simulink model "QP_9B_SimModel"  (R2014a)
settings: Solver=ode45  StartTime=0.0  StopTime=0.2  RelTol=1e-3
values from neighbouring files (symbols this model uses):
  B = mod(B, modulo)    [QP_MD5.m]    (also in QP_SolvePowerFlowEps.m = imag(Y))
  D = generator(:,GEN_D)    [QP_9B_RunModel.m]    (also in QP_MD5.m = C; QP_SimulateSystem.m; QP_SmallSignal.m = generator(:,GEN_D) .* generator(:,3)/100)
  delta0 = deltaState    [QP_9B_RunModel.m]    (also in QP_EXP_SimulateSystem.m = delta1(end,:)'; QP_SimulateSystem.m = delta0'; QP_SmallSignal.m = delta)
  E0_delta = delta0    [QP_9B_RunModel.m]
  G = ss(A, B, C, D)    [QP_HankelSV.m]    (also in QP_SolvePowerFlowEps.m = real(Y))
  H = generator(:,GEN_H)    [QP_9B_RunModel.m]    (also in QP_EXP_MultipleFiltering.m = 0.1; QP_SimulateSystem.m; QP_SmallSignal.m = generator(:,GEN_H) .* generator(:,3)/100)
  Pm = zeros(N_gen,1)    [QP_ClassicalEquilibrium.m]    (also in QP_ClassicalModel.m = [P;zeros(N_node - N_gen, 1)]; QP_SmallSignal.m = P0; QP_dw.m = [P;zeros(N_node - N_gen, 1)])
  RC_State0 = [RC_State.Data(end,1:StateIndex(faultyLine)-1),         RC_State.Data(end,StateIndex(faultyLine)+1:end)]    [QP_9B_RunModel.m]
  SysA = A_PostFault    [QP_9B_RunModel.m]    (also in QP_9B_SSModel.m = SysA([1:RM_State-1,RM_State+1:end],         [1:RM_State-1,RM; QP_ElectricNetwork.m = SysA([1:faultyBus-1, faultyBus+1:end],         [1:faultyBus-; QP_SmallSignal.m = SysA(2:end,2:end))
  SysB = B_PostFault    [QP_9B_RunModel.m]    (also in QP_9B_SSModel.m = SysB([1:RM_State-1,RM_State+1:end],:); QP_ElectricNetwork.m = SysB([1:faultyBus-1, faultyBus+1:end],:))
  SysC = C_PostFault    [QP_9B_RunModel.m]    (also in QP_9B_SSModel.m = SysC(:,[1:RM_State-1,RM_State+1:end]); QP_ElectricNetwork.m = SysC(:,[1:faultyBus-1, faultyBus+1:end]))
  w0 = omegaState    [QP_9B_RunModel.m]    (also in QP_SmallSignal.m = omega)
  XNoisePWR = statePWR([1:StateIndex(faultyLine)-1,              StateIndex(faultyLine)+1:end]) * PWR    [QP_9B_RunModel.m]
  YNoisePWR = outputPWR * PWR    [QP_9B_RunModel.m]
undefined symbols (not defined in the file or in its folder): magnitude
settings Model: Creator=Qiu  LastModifiedBy=qqin
settings DebuggingCC: UnderspecifiedInitializationDetection=Classic  SolverPrmCheckMsg=none  UnconnectedOutputMsg=none  StateNameClashWarn=warning

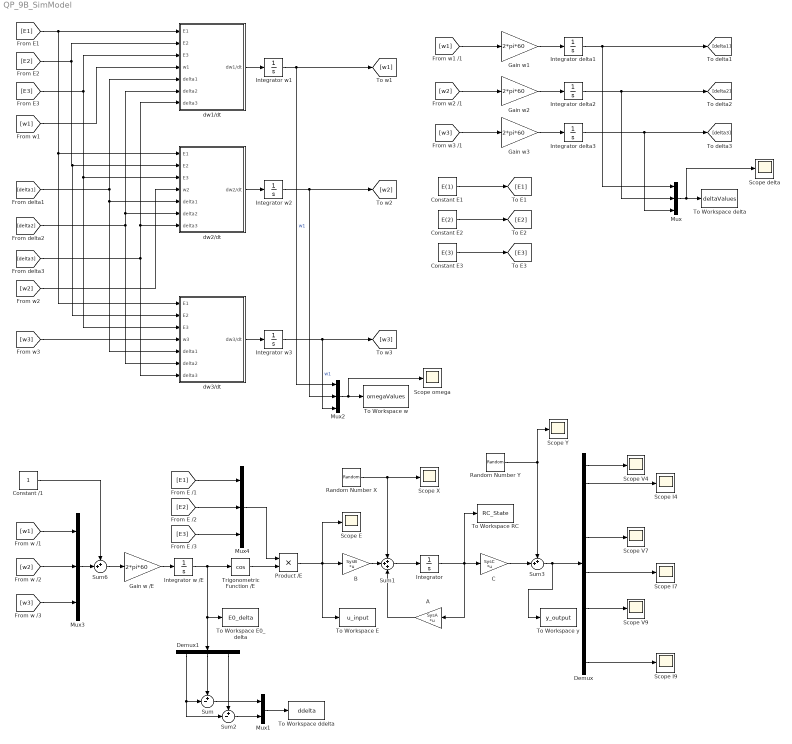
== system QP_9B_SimModel ==
  A : Gain  Gain=SysA  Multiplication=Matrix(K*u)
  B : Gain  Gain=SysB  Multiplication=Matrix(K*u)
  C : Gain  Gain=SysC  Multiplication=Matrix(K*u)
  Constant /1 : Constant
  Constant E1 : Constant  Value=E(1)
  Constant E2 : Constant  Value=E(2)
  Constant E3 : Constant  Value=E(3)
  Demux : Demux  Outputs=12
  Demux1 : Demux  Outputs=3
  Gain w /E : Gain  Gain=2*pi*60
  Gain w1 : Gain  Gain=2*pi*60
  Gain w2 : Gain  Gain=2*pi*60
  Gain w3 : Gain  Gain=2*pi*60
  Integrator : Integrator  InitialCondition=RC_State0
  Integrator delta1 : Integrator  InitialCondition=delta0(1)
  Integrator delta2 : Integrator  InitialCondition=delta0(2)
  Integrator delta3 : Integrator  InitialCondition=delta0(3)
  Integrator w /E : Integrator  InitialCondition=E0_delta
  Integrator w1 : Integrator  InitialCondition=w0(1)
  Integrator w2 : Integrator  InitialCondition=w0(2)
  Integrator w3 : Integrator  InitialCondition=w0(3)
  Mux{,2..4} (4 alike) : Mux  Inputs=3
  Mux1 : Mux  Inputs=2
  Product /E : Product
  Random Number X : RandomNumber  Variance=XNoisePWR  Seed=[round(rand(1)*10000)]  SampleTime=1/60/96
  Random Number Y : RandomNumber  Variance=YNoisePWR  Seed=[round(rand(1)*10000)]  SampleTime=1/60/96
  Scope E : Scope
      settings: MaxDataPoints=50000
  Scope I4 : Scope
      settings: SaveName=ScopeData6  MaxDataPoints=50000
  Scope I7 : Scope
      settings: SaveName=ScopeData7  MaxDataPoints=50000
  Scope I9 : Scope
      settings: SaveName=ScopeData8  MaxDataPoints=50000
  Scope V4 : Scope
      settings: MaxDataPoints=50000
  Scope V7 : Scope
      settings: SaveName=ScopeData2  MaxDataPoints=50000
  Scope V9 : Scope
      settings: SaveName=ScopeData3  MaxDataPoints=50000
  Scope X : Scope
      settings: SaveName=ScopeData10  MaxDataPoints=50000
  Scope Y : Scope
      settings: SaveName=ScopeData9  MaxDataPoints=50000
  Scope delta : Scope
      settings: SaveName=ScopeData4  MaxDataPoints=50000
  Scope omega : Scope
      settings: SaveName=ScopeData5  MaxDataPoints=50000
  Sum : Sum  Inputs=+-|
  Sum1 : Sum  Inputs=+++
  Sum2 : Sum  Inputs=+-|
  Sum3 : Sum  Inputs=++|
  Sum6 : Sum  Inputs=++|
  To Workspace E : ToWorkspace  VariableName=u_input  SaveFormat=Timeseries  SampleTime=-1
      settings: MaxDataPoints=Inf
  To Workspace E0_delta : ToWorkspace  VariableName=E0_delta  SampleTime=-1
      settings: MaxDataPoints=1
  To Workspace RC : ToWorkspace  VariableName=RC_State  SaveFormat=Timeseries  SampleTime=-1
      settings: MaxDataPoints=Inf
  To Workspace ddelta : ToWorkspace  VariableName=ddelta  SaveFormat=Timeseries  SampleTime=-1
      settings: MaxDataPoints=Inf
  To Workspace delta : ToWorkspace  VariableName=deltaValues  SampleTime=-1
      settings: MaxDataPoints=1
  To Workspace w : ToWorkspace  VariableName=omegaValues  SaveFormat=Timeseries  SampleTime=-1
      settings: MaxDataPoints=Inf
  To Workspace y : ToWorkspace  VariableName=y_output  SaveFormat=Timeseries  SampleTime=-1
      settings: MaxDataPoints=Inf
  Trigonometric Function /E : Trigonometry  Operator=cos
  dw1/dt : Subsystem
  dw2/dt : Subsystem
  dw3/dt : Subsystem
  wires:
  Integrator w1/1 -> Mux2/1, [w1]  "w1"
  Gain w1/1 -> Integrator delta1/1
  Integrator delta1/1 -> Mux/1, [delta1]
  [w1] -> Gain w1/1
  Gain w2/1 -> Integrator delta2/1
  [w2] -> Gain w2/1
  Gain w3/1 -> Integrator delta3/1
  [w3] -> Gain w3/1
  Integrator delta2/1 -> [delta2], Mux/2
  Integrator delta3/1 -> [delta3], Mux/3
  Constant E1/1 -> [E1]
  Constant E2/1 -> [E2]
  Constant E3/1 -> [E3]
  dw1/dt/1(dw1/dt) -> Integrator w1/1
  Integrator w2/1 -> Mux2/2, [w2]
  dw2/dt/1(dw2/dt) -> Integrator w2/1
  Integrator w3/1 -> Mux2/3, [w3]  "w1"
  dw3/dt/1(dw3/dt) -> Integrator w3/1
  Mux/1 -> Scope delta/1, To Workspace delta/1
  [w2] -> dw2/dt/4(w2)
  [w3] -> dw3/dt/4(w3)
  [E1] -> dw3/dt/1(E1), dw2/dt/1(E1), dw1/dt/1(E1)
  [E2] -> dw3/dt/2(E2), dw2/dt/2(E2), dw1/dt/2(E2)
  [E3] -> dw3/dt/3(E3), dw2/dt/3(E3), dw1/dt/3(E3)
  [delta1] -> dw1/dt/5(delta1), dw3/dt/5(delta1), dw2/dt/5(delta1)
  [delta2] -> dw3/dt/6(delta2), dw1/dt/6(delta2), dw2/dt/6(delta2)
  [delta3] -> dw3/dt/7(delta3), dw1/dt/7(delta3), dw2/dt/7(delta3)
  [w1] -> dw1/dt/4(w1)
  Mux2/1 -> Scope omega/1, To Workspace w/1
  Sum1/1 -> Integrator/1
  Integrator/1 -> To Workspace RC/1, A/1, C/1
  Product /E/1 -> To Workspace E/1, Scope E/1, B/1
  Demux/1 -> Scope V4/1
  Demux/5 -> Scope V7/1
  Demux/9 -> Scope V9/1
  Trigonometric Function /E/1 -> Product /E/2
  Integrator w /E/1 -> Demux1/1, To Workspace E0_delta/1, Trigonometric Function /E/1
  Constant /1/1 -> Sum6/1
  Sum6/1 -> Gain w /E/1
  Demux/2 -> Scope I4/1
  Demux/12 -> Scope I9/1
  Demux/7 -> Scope I7/1
  Gain w /E/1 -> Integrator w /E/1
  Mux3/1 -> Sum6/2
  [w1] -> Mux3/1
  [w2] -> Mux3/2
  [w3] -> Mux3/3
  [E1] -> Mux4/1
  [E2] -> Mux4/2
  [E3] -> Mux4/3
  Mux4/1 -> Product /E/1
  Demux1/1 -> Sum/2, Sum2/2
  Demux1/2 -> Sum/1
  Demux1/3 -> Sum2/1
  Mux1/1 -> To Workspace ddelta/1
  Sum/1 -> Mux1/1
  Sum2/1 -> Mux1/2
  B/1 -> Sum1/2
  A/1 -> Sum1/3
  Random Number X/1 -> Scope X/1, Sum1/1
  Random Number Y/1 -> Scope Y/1, Sum3/1
  C/1 -> Sum3/2
  Sum3/1 -> To Workspace y/1, Demux/1

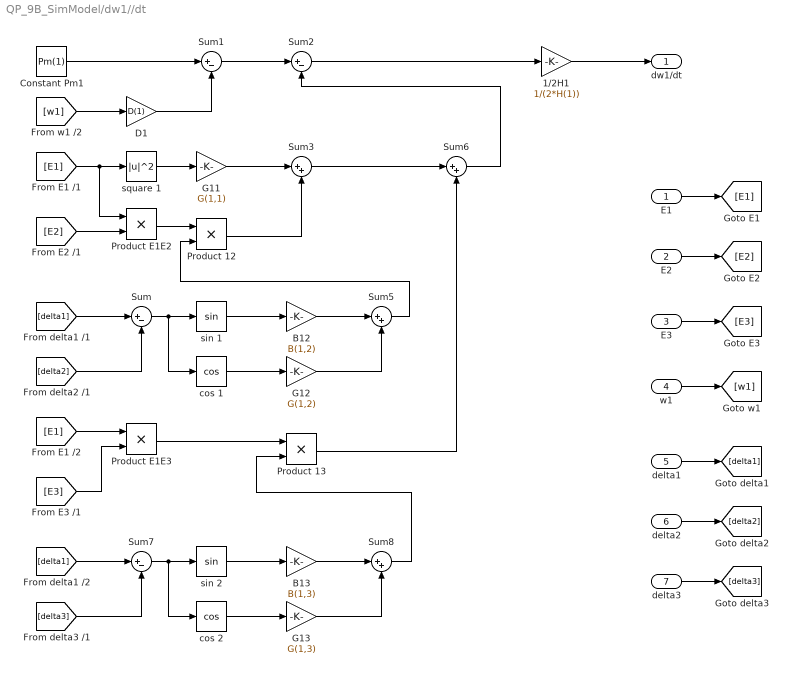
== system QP_9B_SimModel/dw1//dt ==
  E1 : Inport
  E2 : Inport  Port=2
  E3 : Inport  Port=3
  w1 : Inport  Port=4
  delta1 : Inport  Port=5
  delta2 : Inport  Port=6
  delta3 : Inport  Port=7
  1/2H1 : Gain  Gain=1/(2*H(1))
  B12 : Gain  Gain=B(1,2)
  B13 : Gain  Gain=B(1,3)
  Constant Pm1 : Constant  Value=Pm(1)
  D1 : Gain  Gain=D(1)
  G11 : Gain  Gain=G(1,1)
  G12 : Gain  Gain=G(1,2)
  G13 : Gain  Gain=G(1,3)
  Product 12 : Product
  Product 13 : Product
  Product E1E2 : Product
  Product E1E3 : Product
  Sum{,1..2,7} (4 alike) : Sum  Inputs=|+-
  Sum{3,5..6,8} (4 alike) : Sum  Inputs=|++
  cos 1 : Trigonometry  Operator=cos
  cos 2 : Trigonometry  Operator=cos
  sin 1 : Trigonometry
  sin 2 : Trigonometry
  square 1 : Math  Operator=magnitude^2  SaturateOnIntegerOverflow=on
  dw1/dt : Outport
  wires:
  G11/1 -> Sum3/1
  Sum3/1 -> Sum6/1
  Product 12/1 -> Sum3/2
  [delta2] -> Sum/2
  Product E1E2/1 -> Product 12/1
  sin 1/1 -> B12/1
  G12/1 -> Sum5/2
  [E2] -> Product E1E2/2
  [E1] -> Product E1E3/1
  B12/1 -> Sum5/1
  Sum8/1 -> Product 13/2
  Product 13/1 -> Sum6/2
  Sum2/1 -> 1/2H1/1
  Sum6/1 -> Sum2/2
  Sum7/1 -> cos 2/1, sin 2/1
  [delta1] -> Sum7/1
  sin 2/1 -> B13/1
  [delta3] -> Sum7/2
  cos 2/1 -> G13/1
  B13/1 -> Sum8/1
  G13/1 -> Sum8/2
  1/2H1/1 -> dw1/dt/1
  [delta1] -> Sum/1
  square 1/1 -> G11/1
  Constant Pm1/1 -> Sum1/1
  Sum1/1 -> Sum2/1
  D1/1 -> Sum1/2
  Product E1E3/1 -> Product 13/1
  Sum/1 -> cos 1/1, sin 1/1
  [E3] -> Product E1E3/2
  [w1] -> D1/1
  cos 1/1 -> G12/1
  [E1] -> Product E1E2/1, square 1/1
  Sum5/1 -> Product 12/2
  E1/1 -> [E1]
  E2/1 -> [E2]
  E3/1 -> [E3]
  w1/1 -> [w1]
  delta1/1 -> [delta1]
  delta2/1 -> [delta2]
  delta3/1 -> [delta3]

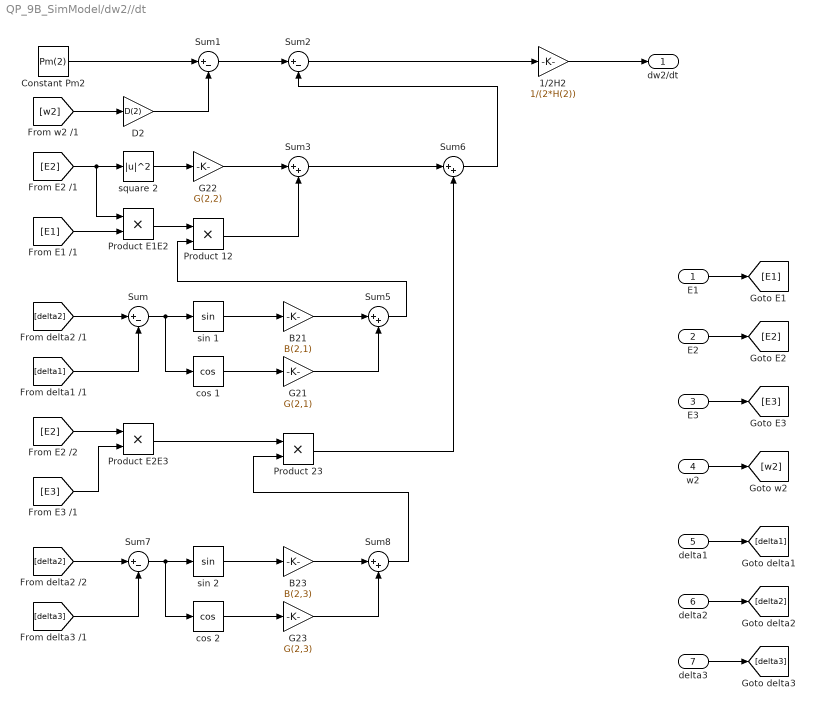
== system QP_9B_SimModel/dw2//dt ==
  E1 : Inport
  E2 : Inport  Port=2
  E3 : Inport  Port=3
  w2 : Inport  Port=4
  delta1 : Inport  Port=5
  delta2 : Inport  Port=6
  delta3 : Inport  Port=7
  1/2H2 : Gain  Gain=1/(2*H(2))
  B21 : Gain  Gain=B(2,1)
  B23 : Gain  Gain=B(2,3)
  Constant Pm2 : Constant  Value=Pm(2)
  D2 : Gain  Gain=D(2)
  G21 : Gain  Gain=G(2,1)
  G22 : Gain  Gain=G(2,2)
  G23 : Gain  Gain=G(2,3)
  Product 12 : Product
  Product 23 : Product
  Product E1E2 : Product
  Product E2E3 : Product
  Sum{,1..2,7} (4 alike) : Sum  Inputs=|+-
  Sum{3,5..6,8} (4 alike) : Sum  Inputs=|++
  cos 1 : Trigonometry  Operator=cos
  cos 2 : Trigonometry  Operator=cos
  sin 1 : Trigonometry
  sin 2 : Trigonometry
  square 2 : Math  Operator=magnitude^2  SaturateOnIntegerOverflow=on
  dw2/dt : Outport
  wires:
  G22/1 -> Sum3/1
  Sum3/1 -> Sum6/1
  Product 12/1 -> Sum3/2
  Product E1E2/1 -> Product 12/1
  sin 1/1 -> B21/1
  G21/1 -> Sum5/2
  [E1] -> Product E1E2/2
  [E2] -> Product E2E3/1
  B21/1 -> Sum5/1
  Sum8/1 -> Product 23/2
  Product 23/1 -> Sum6/2
  Sum2/1 -> 1/2H2/1
  Sum6/1 -> Sum2/2
  Sum7/1 -> cos 2/1, sin 2/1
  [delta2] -> Sum7/1
  sin 2/1 -> B23/1
  [delta3] -> Sum7/2
  cos 2/1 -> G23/1
  B23/1 -> Sum8/1
  G23/1 -> Sum8/2
  1/2H2/1 -> dw2/dt/1
  square 2/1 -> G22/1
  Constant Pm2/1 -> Sum1/1
  Sum1/1 -> Sum2/1
  D2/1 -> Sum1/2
  Product E2E3/1 -> Product 23/1
  Sum/1 -> cos 1/1, sin 1/1
  [E3] -> Product E2E3/2
  [w2] -> D2/1
  cos 1/1 -> G21/1
  [E2] -> Product E1E2/1, square 2/1
  Sum5/1 -> Product 12/2
  [delta2] -> Sum/1
  [delta1] -> Sum/2
  E1/1 -> [E1]
  E2/1 -> [E2]
  E3/1 -> [E3]
  w2/1 -> [w2]
  delta1/1 -> [delta1]
  delta2/1 -> [delta2]
  delta3/1 -> [delta3]

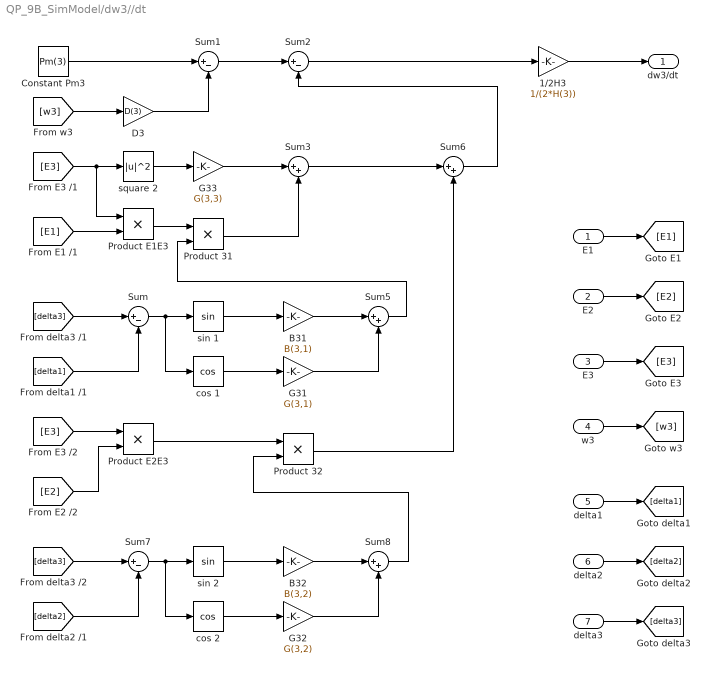
== system QP_9B_SimModel/dw3//dt ==
  E1 : Inport
  E2 : Inport  Port=2
  E3 : Inport  Port=3
  w3 : Inport  Port=4
  delta1 : Inport  Port=5
  delta2 : Inport  Port=6
  delta3 : Inport  Port=7
  1/2H3 : Gain  Gain=1/(2*H(3))
  B31 : Gain  Gain=B(3,1)
  B32 : Gain  Gain=B(3,2)
  Constant Pm3 : Constant  Value=Pm(3)
  D3 : Gain  Gain=D(3)
  G31 : Gain  Gain=G(3,1)
  G32 : Gain  Gain=G(3,2)
  G33 : Gain  Gain=G(3,3)
  Product 31 : Product
  Product 32 : Product
  Product E1E3 : Product
  Product E2E3 : Product
  Sum{,1..2,7} (4 alike) : Sum  Inputs=|+-
  Sum{3,5..6,8} (4 alike) : Sum  Inputs=|++
  cos 1 : Trigonometry  Operator=cos
  cos 2 : Trigonometry  Operator=cos
  sin 1 : Trigonometry
  sin 2 : Trigonometry
  square 2 : Math  Operator=magnitude^2  SaturateOnIntegerOverflow=on
  dw3/dt : Outport
  wires:
  G33/1 -> Sum3/1
  Sum3/1 -> Sum6/1
  Product 31/1 -> Sum3/2
  Product E1E3/1 -> Product 31/1
  sin 1/1 -> B31/1
  G31/1 -> Sum5/2
  [E1] -> Product E1E3/2
  [E3] -> Product E2E3/1
  B31/1 -> Sum5/1
  Sum8/1 -> Product 32/2
  Product 32/1 -> Sum6/2
  Sum2/1 -> 1/2H3/1
  Sum6/1 -> Sum2/2
  Sum7/1 -> cos 2/1, sin 2/1
  [delta3] -> Sum7/1
  sin 2/1 -> B32/1
  [delta2] -> Sum7/2
  cos 2/1 -> G32/1
  B32/1 -> Sum8/1
  G32/1 -> Sum8/2
  1/2H3/1 -> dw3/dt/1
  square 2/1 -> G33/1
  Constant Pm3/1 -> Sum1/1
  Sum1/1 -> Sum2/1
  D3/1 -> Sum1/2
  Product E2E3/1 -> Product 32/1
  Sum/1 -> cos 1/1, sin 1/1
  [E2] -> Product E2E3/2
  [w3] -> D3/1
  cos 1/1 -> G31/1
  [E3] -> Product E1E3/1, square 2/1
  Sum5/1 -> Product 31/2
  [delta3] -> Sum/1
  [delta1] -> Sum/2
  E1/1 -> [E1]
  E2/1 -> [E2]
  E3/1 -> [E3]
  w3/1 -> [w3]
  delta1/1 -> [delta1]
  delta2/1 -> [delta2]
  delta3/1 -> [delta3]
